simulink model "LQGNonLinearFunction"  (R2019a)
settings: Solver=VariableStepAuto  StartTime=0.0  StopTime=100  RelTol=1e-3
values from neighbouring files (symbols this model uses):
  ALI = [ 0, 1,         0, 0,        0, 0 ... (first row only)    [LQRControlLinearised.m]    (also in LyapunovIndirectMethod.m; ObservabilityCheck.m)
  BLI = [0 ... (first row only)    [LQRControlLinearised.m]    (also in LyapunovIndirectMethod.m; ObservabilityCheck.m)
  C = [1 0 0 0 0 0 ... (first row only)    [ControllabilityCheck.m]    (also in LQGControlLinear.m = [1 0 0 0 0 0]; LQRControlLinearised.m; LQRControlNonLinear.m; LyapunovIndirectMethod.m)
  D = zeros(3,1)    [ControllabilityCheck.m]    (also in LQGControlLinear.m = 0; LQRControlLinearised.m = zeros(1,1); LQRControlNonLinear.m = [0]; LyapunovIndirectMethod.m = zeros(1,1))
undefined symbols (not defined in the file or in its folder): Continuous, KLI, Time
libraries: ctrlSharedLib x1
settings Model: Creator=Prasheel Renkuntla  LastModifiedBy=Prasheel Renkuntla

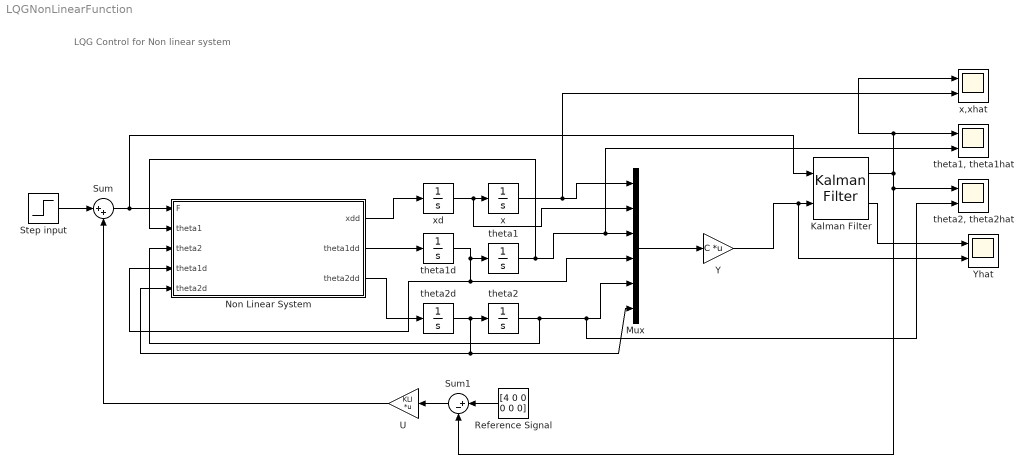
== system LQGNonLinearFunction ==
  note: LQG Control for Non linear system
  "Kalman Filter " : ctrlSharedLib/Kalman Filter  TimeDomain=Continuous-Time  UseCurrentEstimator=on  ModelSource=Individual A, B, C, D matrices  ModelSourceVariable=ss(0.95,1,1,0,1)  A=ALI  B=BLI  C=C  D=D  NumberOfStates=1  NumberOfInputs=1  NumberOfOutputs=1  InitialEstimateSource=Dialog  X0=[4; 0; 0.1; 0; 0.1; 0]  P0=10  UseK=off  UseGH=off  NumberOfProcessNoiseInputs=1  G=1  TimeInvariantG=on  H=0  TimeInvariantH=on  Q=1  TimeInvariantQ=on  R=1  TimeInvariantR=on  N=0  TimeInvariantN=on  AddInputPort=on  AddEnablePort=off  OutputEstimatedY=on  OutputP=off  Ts=-1
      settings: SourceProductBaseCode=CT
  Mux : Mux  Inputs=6
  "Non Linear System " : MATLAB Function  TreatAsAtomicUnit=on
  Reference Signal : Constant  Value=[4 0 0 0 0 0]
  Step input : Step  SampleTime=0
  Sum : Sum  Inputs=|++
  Sum1 : Sum  Inputs=|+-
  U : Gain  Gain=KLI  Multiplication=Matrix(K*u)
  Y : Gain  Gain=C  Multiplication=Matrix(K*u)
  Yhat : Scope  NumInputPorts=2
  theta1 : Integrator
  "theta1, theta1hat" : Scope  NumInputPorts=2
  theta1d : Integrator
  theta2 : Integrator
  "theta2, theta2hat" : Scope  NumInputPorts=2
  theta2d : Integrator
  x : Integrator
  x,xhat : Scope  NumInputPorts=2
  xd : Integrator
  wires:
  Step input/1 -> Sum/1
  Sum/1 -> "Kalman Filter "/1, "Non Linear System "/1(F)
  "Non Linear System "/1(xdd) -> xd/1
  xd/1 -> Mux/2, x/1
  theta1d/1 -> "Non Linear System "/4(theta1d), Mux/4, theta1/1
  theta2d/1 -> "Non Linear System "/5(theta2d), Mux/6, theta2/1
  "Non Linear System "/2(theta1dd) -> theta1d/1
  "Non Linear System "/3(theta2dd) -> theta2d/1
  x/1 -> x,xhat/2, Mux/1
  theta1/1 -> "Non Linear System "/2(theta1), "theta1, theta1hat"/2, Mux/3
  theta2/1 -> "Non Linear System "/3(theta2), "theta2, theta2hat"/2, Mux/5
  Mux/1 -> Y/1
  Y/1 -> Yhat/2, "Kalman Filter "/2
  "Kalman Filter "/2 -> Yhat/1
  Reference Signal/1 -> Sum1/1
  Sum1/1 -> U/1
  U/1 -> Sum/2
  "Kalman Filter "/1 -> "theta2, theta2hat"/1, Sum1/2, x,xhat/1, "theta1, theta1hat"/1

== matlab function LQGNonLinearFunction/Non Linear System  ==
  data: F input; xdd output; theta1 input; theta2 input; theta1d input; theta2d input; theta1dd output; theta2dd output
function [xdd, theta1dd, theta2dd] = LQGNL(F, theta1, theta2, theta1d, theta2d)
M = 1000;
m1 = 100;
m2 = 100;
l1 = 20;
l2 = 10;
g =9.8;
xdd = (F - m1*g*sind(theta1)*cosd(theta1) - m2*g*sind(theta2)*cosd(theta2) - m1*l1*theta1d*theta1d*sind(theta1) - m2*l2*theta2d*theta2d*sind(theta2))/(M + m1*sind(theta1)*sind(theta1) + m2*sind(theta2)*sind(theta2));
theta1dd = (xdd*cosd(theta1) - g*(sind(theta1)))/(l1);
theta2dd = (xdd*cosd(theta2) - g*(sind(theta2)))/(l2);
end
